simulink model "ExtensionSimulation1var_5"  (R2017b)
settings: Solver=VariableStepAuto  StartTime=0.0  StopTime=60  RelTol=1e-3  EnableMultiTasking=on
values from neighbouring files (symbols this model uses):
  CHNoise = 1e-05    [Extension 1 Variables.mat]    (also in PlotChannelDiscrete.m = 1e-10; PlotChannelsExt.m = 0.0001; SelectivityFunction.m = 0.001)
  nu_gpe = 1    [Extension 1 Variables.mat]
  nu_gpi = 1    [Extension 1 Variables.mat]
  nu_stn = 1    [Extension 1 Variables.mat]
  nu_str = 1    [Extension 1 Variables.mat]
  teta = 0.02    [Extension 1 Variables.mat]
  w_e = 0.9    [Extension 1 Variables.mat]    (also in PlotChannelsExt.m = 1)
  w_g = 1    [Extension 1 Variables.mat]
  w_inh = 0    [Extension 1 Variables.mat]    (also in PlotChannelsExt.m = 0.1)
  w_minus = 1    [Extension 1 Variables.mat]    (also in PlotChannelsExt.m = 1.05)
  w_plus = 0.9    [Extension 1 Variables.mat]    (also in PlotChannelsExt.m = 1)
  w_s = 1    [Extension 1 Variables.mat]    (also in PlotChannelsExt.m)
  w_t = 0.9    [Extension 1 Variables.mat]    (also in PlotChannelsExt.m = 1)
undefined symbols (not defined in the file or in its folder): sigbuilder_block
libraries: fuzblock x25, simulink x8
settings Model: Creator=User  LastModifiedBy=acaso
settings DataIOCC: LimitDataPoints=on
settings OptimizationCC: LifeSpan=inf
settings DebuggingCC: AllowSymbolicDim=off  SFUnexpectedBacktrackingDiag=warning  SFNoUnconditionalDefaultTransitionDiag=warning  SFExecutionAtInitializationDiag=none
settings ModelReferenceCC: PropagateSignalLabelsOutOfModel=off
settings CodeAppCC: StateflowObjectComments=on
settings GRTTargetCC: TargetLangStandard=C89/C90 (ANSI)
settings ConfigComp: CovMetricSettings=dw  CovHtmlReporting=on  CovSaveCumulativeToWorkspaceVar=on  CovSaveSingleToWorkspaceVar=on  CovExternalEMLEnable=off

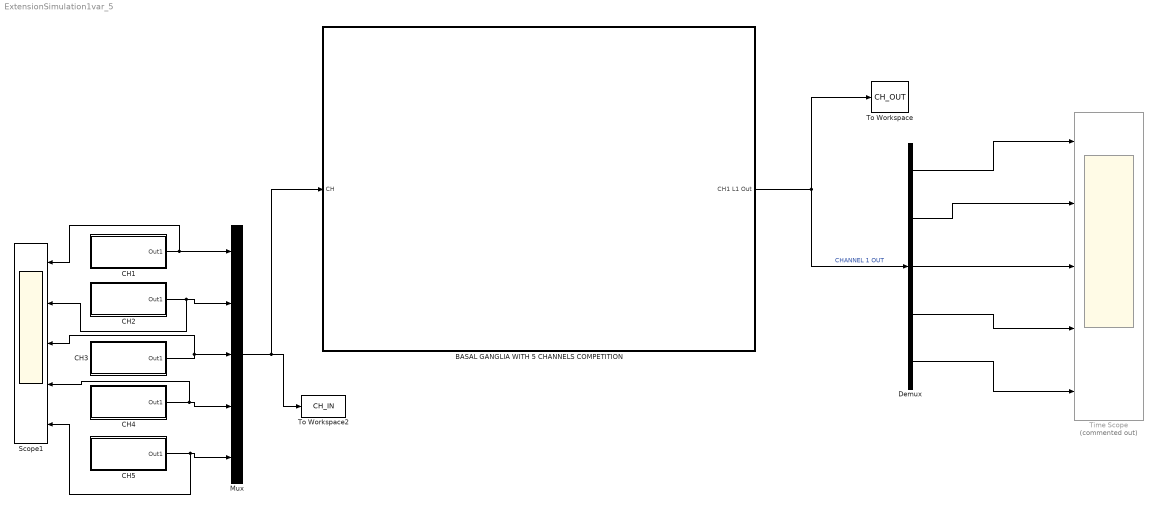
== system ExtensionSimulation1var_5 ==
  BASAL GANGLIA WITH 5 CHANNELS COMPETITION : Subsystem
  "CH1 " : Subsystem
  CH2 : Subsystem
  "CH3 " : Subsystem
  "CH4 " : Subsystem
  "CH5 " : Subsystem
  Demux : Demux  Outputs=5
  Mux : Mux  Inputs=5
  Scope1 : Scope  NumInputPorts=5
  Time Scope : Scope  Commented=on  NumInputPorts=5
  To Workspace : ToWorkspace  VariableName=CH_OUT  SaveFormat=Timeseries  SampleTime=0.1
      settings: Save2DSignal=2-D array (concatenate along first dimension)
  To Workspace2 : ToWorkspace  VariableName=CH_IN  SaveFormat=Timeseries  SampleTime=0.1
  wires:
  BASAL GANGLIA WITH 5 CHANNELS COMPETITION/1(CH1 L1 Out) -> Demux/1, To Workspace/1  "CHANNEL 1 OUT"
  "CH1 "/1(Out1) -> Scope1/1, Mux/1
  "CH3 "/1(Out1) -> Scope1/3, Mux/3
  "CH4 "/1(Out1) -> Scope1/4, Mux/4
  "CH5 "/1(Out1) -> Scope1/5, Mux/5
  Mux/1 -> BASAL GANGLIA WITH 5 CHANNELS COMPETITION/1("CH "), To Workspace2/1
  Demux/1 -> Time Scope/1
  Demux/2 -> Time Scope/2
  Demux/3 -> Time Scope/3
  Demux/4 -> Time Scope/4
  Demux/5 -> Time Scope/5
  CH2/1(Out1) -> Scope1/2, Mux/2

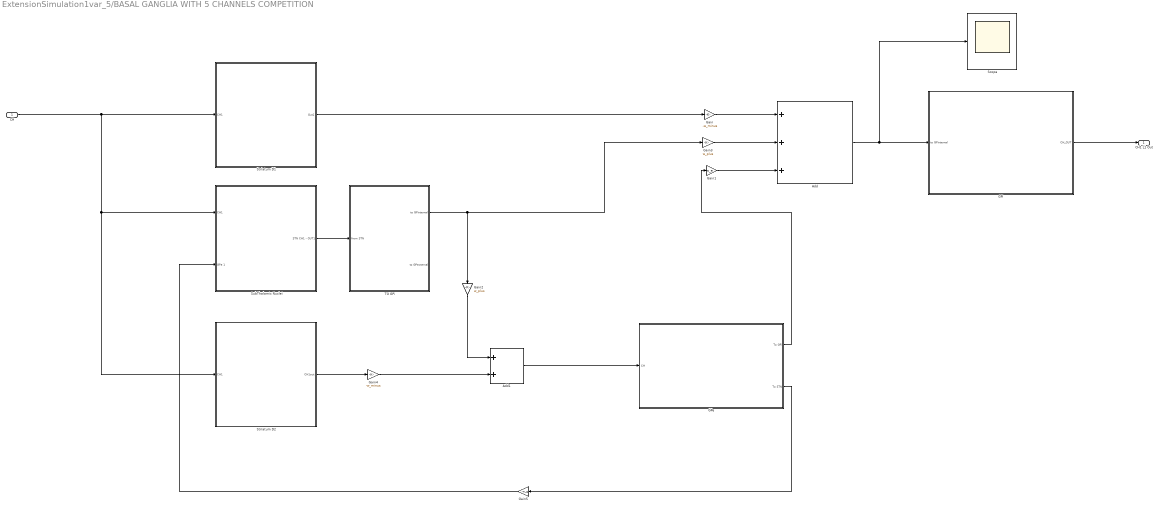
== system ExtensionSimulation1var_5/BASAL GANGLIA WITH 5 CHANNELS COMPETITION ==
  "CH " : Inport
  Add : Sum  Inputs=3
  Add1 : Sum  Inputs=2
  GPe : Subsystem  TreatAsAtomicUnit=on
  GPi : Subsystem
  Gain : Gain  Gain=-w_minus
  Gain1 : Gain  Gain=w_e
  Gain2 : Gain  Gain=w_plus
  Gain3 : Gain  Gain=w_plus
  Gain4 : Gain  Gain=-w_minus
  Gain5 : Gain  Gain=-w_g
  Scope : Scope
  "Striatum D1 " : Subsystem
  Striatum D2 : Subsystem
  SubThalamic Nuclei : Subsystem
  TO GPi : Subsystem
  CH1 L1 Out : Outport
  wires:
  TO GPi/1(to GPinternal) -> Gain2/1, Gain3/1
  GPi/1("CH_OUT ") -> CH1 L1 Out/1
  "CH "/1 -> Striatum D2/1(CH1), SubThalamic Nuclei/1(CH1), "Striatum D1 "/1(CH1)
  "Striatum D1 "/1(Out1) -> Gain/1
  SubThalamic Nuclei/1(STN CH1 - OUT1) -> TO GPi/1("from STN ")
  GPe/1(To GPi) -> Gain1/1
  Gain/1 -> Add/1
  Gain3/1 -> Add/2
  Gain1/1 -> Add/3
  Striatum D2/1(CH1out) -> Gain4/1
  Gain2/1 -> Add1/1
  Gain4/1 -> Add1/2
  Add1/1 -> GPe/1(CH)
  GPe/2(To STN) -> Gain5/1
  Gain5/1 -> SubThalamic Nuclei/2(GPe 1)
  Add/1 -> GPi/1("to GPinternal "), Scope/1

== system ExtensionSimulation1var_5/CH1  ==
  Add : Sum
  Band-Limited White Noise : simulink/Sources/Band-Limited White Noise  Cov=[CHNoise]  Ts=0.1  seed=[23341]
  "CHANNEL1 IN " : Subsystem  Tag=STV Subsys  LoadFcn=sigbuilder_block('load');  StartFcn=sigbuilder_block('start');  StopFcn=sigbuilder_block('stop');  ClipboardFcn=sigbuilder_block('clipboard');  mask(Sigbuilder block){tuvar=[0:10]}
      mask help: Simulink:masks:SigbuilderBlock_MD
      mask init:
      | if ~strcmp(get_param(bdroot(gcbh),'SimulationStatus'),'stopped') tuvar = sigbuilder_block('maskInit'); end
      settings: CopyFcn=sigbuilder_block('copy');  DeleteFcn=sigbuilder_block('delete');  ModelCloseFcn=sigbuilder_block('modelClose');  PreSaveFcn=sigbuilder_block('preSave');  PauseFcn=sigbuilder_block('pause');  ContinueFcn=sigbuilder_block('continue');  NameChangeFcn=sigbuilder_block('namechange');  OpenFcn=sigbuilder_block('open',[5.4 5.4 1141.2 580.8 ]);  CloseFcn=sigbuilder_block('close');
      mask Display: plot(0, 0, 100, 100,[2, 2, 32, 32, 2], [68, 8, 8, 68, 68],[32, 2], [38, 38], [32, 19, 2],[53, 60, 44], [32, 17, 17, 2],[16, 16, 31, 31]);txt = getActiveGroup(gcbh);text(2, 100, txt,'verticalAlignment', 'top');
  Out1 : Outport
  wires:
  Band-Limited White Noise/1 -> Add/2
  Add/1 -> Out1/1
  "CHANNEL1 IN "/1(Signal 1) -> Add/1

== system ExtensionSimulation1var_5/CH2 ==
  Add : Sum
  Band-Limited White Noise : simulink/Sources/Band-Limited White Noise  Cov=[CHNoise]  Ts=0.1  seed=[23341]
  "CHANNEL2 IN " : Subsystem  Tag=STV Subsys  LoadFcn=sigbuilder_block('load');  StartFcn=sigbuilder_block('start');  StopFcn=sigbuilder_block('stop');  ClipboardFcn=sigbuilder_block('clipboard');  mask(Sigbuilder block){tuvar=[0:10]}
      mask help: Simulink:masks:SigbuilderBlock_MD
      mask init:
      | if ~strcmp(get_param(bdroot(gcbh),'SimulationStatus'),'stopped') tuvar = sigbuilder_block('maskInit'); end
      settings: CopyFcn=sigbuilder_block('copy');  DeleteFcn=sigbuilder_block('delete');  ModelCloseFcn=sigbuilder_block('modelClose');  PreSaveFcn=sigbuilder_block('preSave');  PauseFcn=sigbuilder_block('pause');  ContinueFcn=sigbuilder_block('continue');  NameChangeFcn=sigbuilder_block('namechange');  OpenFcn=sigbuilder_block('open',[268.8 5.4 877.8 580.8 ]);  CloseFcn=sigbuilder_block('close');
      mask Display: plot(0, 0, 100, 100,[2, 2, 32, 32, 2], [68, 8, 8, 68, 68],[32, 2], [38, 38], [32, 19, 2],[53, 60, 44], [32, 17, 17, 2],[16, 16, 31, 31]);txt = getActiveGroup(gcbh);text(2, 100, txt,'verticalAlignment', 'top');
  Out1 : Outport
  wires:
  Band-Limited White Noise/1 -> Add/2
  Add/1 -> Out1/1
  "CHANNEL2 IN "/1(Signal 1) -> Add/1

== system ExtensionSimulation1var_5/CH3  ==
  Add : Sum
  Band-Limited White Noise : simulink/Sources/Band-Limited White Noise  Cov=[CHNoise]  Ts=0.1  seed=[23341]
  "CHANNEL2 IN " : Subsystem  Tag=STV Subsys  LoadFcn=sigbuilder_block('load');  StartFcn=sigbuilder_block('start');  StopFcn=sigbuilder_block('stop');  ClipboardFcn=sigbuilder_block('clipboard');  mask(Sigbuilder block){tuvar=[0:10]}
      mask help: Simulink:masks:SigbuilderBlock_MD
      mask init:
      | if ~strcmp(get_param(bdroot(gcbh),'SimulationStatus'),'stopped') tuvar = sigbuilder_block('maskInit'); end
      settings: CopyFcn=sigbuilder_block('copy');  DeleteFcn=sigbuilder_block('delete');  ModelCloseFcn=sigbuilder_block('modelClose');  PreSaveFcn=sigbuilder_block('preSave');  PauseFcn=sigbuilder_block('pause');  ContinueFcn=sigbuilder_block('continue');  NameChangeFcn=sigbuilder_block('namechange');  OpenFcn=sigbuilder_block('open',[5.4 5.4 1141.2 580.8 ]);  CloseFcn=sigbuilder_block('close');
      mask Display: plot(0, 0, 100, 100,[2, 2, 32, 32, 2], [68, 8, 8, 68, 68],[32, 2], [38, 38], [32, 19, 2],[53, 60, 44], [32, 17, 17, 2],[16, 16, 31, 31]);txt = getActiveGroup(gcbh);text(2, 100, txt,'verticalAlignment', 'top');
  Out1 : Outport
  wires:
  Band-Limited White Noise/1 -> Add/2
  Add/1 -> Out1/1
  "CHANNEL2 IN "/3(Signal 2) -> Add/1

== system ExtensionSimulation1var_5/CH4  ==
  Add : Sum
  Band-Limited White Noise : simulink/Sources/Band-Limited White Noise  Cov=[CHNoise]  Ts=0.1  seed=[23341]
  "CHANNEL2 IN " : Subsystem  Tag=STV Subsys  LoadFcn=sigbuilder_block('load');  StartFcn=sigbuilder_block('start');  StopFcn=sigbuilder_block('stop');  ClipboardFcn=sigbuilder_block('clipboard');  mask(Sigbuilder block){tuvar=[0:10]}
      mask help: Simulink:masks:SigbuilderBlock_MD
      mask init:
      | if ~strcmp(get_param(bdroot(gcbh),'SimulationStatus'),'stopped') tuvar = sigbuilder_block('maskInit'); end
      settings: CopyFcn=sigbuilder_block('copy');  DeleteFcn=sigbuilder_block('delete');  ModelCloseFcn=sigbuilder_block('modelClose');  PreSaveFcn=sigbuilder_block('preSave');  PauseFcn=sigbuilder_block('pause');  ContinueFcn=sigbuilder_block('continue');  NameChangeFcn=sigbuilder_block('namechange');  OpenFcn=sigbuilder_block('open',[5.4 5.4 1141.2 580.8 ]);  CloseFcn=sigbuilder_block('close');
      mask Display: plot(0, 0, 100, 100,[2, 2, 32, 32, 2], [68, 8, 8, 68, 68],[32, 2], [38, 38], [32, 19, 2],[53, 60, 44], [32, 17, 17, 2],[16, 16, 31, 31]);txt = getActiveGroup(gcbh);text(2, 100, txt,'verticalAlignment', 'top');
  Out1 : Outport
  wires:
  Band-Limited White Noise/1 -> Add/2
  Add/1 -> Out1/1
  "CHANNEL2 IN "/2(Signal 2) -> Add/1

== system ExtensionSimulation1var_5/CH5  ==
  Add : Sum
  Band-Limited White Noise : simulink/Sources/Band-Limited White Noise  Cov=[CHNoise]  Ts=0.1  seed=[23341]
  "CHANNEL2 IN " : Subsystem  Tag=STV Subsys  LoadFcn=sigbuilder_block('load');  StartFcn=sigbuilder_block('start');  StopFcn=sigbuilder_block('stop');  ClipboardFcn=sigbuilder_block('clipboard');  mask(Sigbuilder block){tuvar=[0:10]}
      mask help: Simulink:masks:SigbuilderBlock_MD
      mask init:
      | if ~strcmp(get_param(bdroot(gcbh),'SimulationStatus'),'stopped') tuvar = sigbuilder_block('maskInit'); end
      settings: CopyFcn=sigbuilder_block('copy');  DeleteFcn=sigbuilder_block('delete');  ModelCloseFcn=sigbuilder_block('modelClose');  PreSaveFcn=sigbuilder_block('preSave');  PauseFcn=sigbuilder_block('pause');  ContinueFcn=sigbuilder_block('continue');  NameChangeFcn=sigbuilder_block('namechange');  OpenFcn=sigbuilder_block('open',[5.4 5.4 1141.2 580.8 ]);  CloseFcn=sigbuilder_block('close');
      mask Display: plot(0, 0, 100, 100,[2, 2, 32, 32, 2], [68, 8, 8, 68, 68],[32, 2], [38, 38], [32, 19, 2],[53, 60, 44], [32, 17, 17, 2],[16, 16, 31, 31]);txt = getActiveGroup(gcbh);text(2, 100, txt,'verticalAlignment', 'top');
  Out1 : Outport
  wires:
  Band-Limited White Noise/1 -> Add/2
  Add/1 -> Out1/1
  "CHANNEL2 IN "/2(Signal 2) -> Add/1

== system ExtensionSimulation1var_5/BASAL GANGLIA WITH 5 CHANNELS COMPETITION/GPe ==
  CH : Inport
  GPe CH1 : Subsystem
  To GPi : Outport
  To STN : Outport  Port=2
  wires:
  CH/1 -> GPe CH1/1(In)
  GPe CH1/1(To GPi) -> To GPi/1
  GPe CH1/2(To STN) -> To STN/1

== system ExtensionSimulation1var_5/BASAL GANGLIA WITH 5 CHANNELS COMPETITION/GPi ==
  "to GPinternal " : Inport
  GPinternal : Subsystem
  "CH_OUT " : Outport
  wires:
  "to GPinternal "/1 -> GPinternal/1("to GPinternal ")
  GPinternal/1(To Thal) -> "CH_OUT "/1

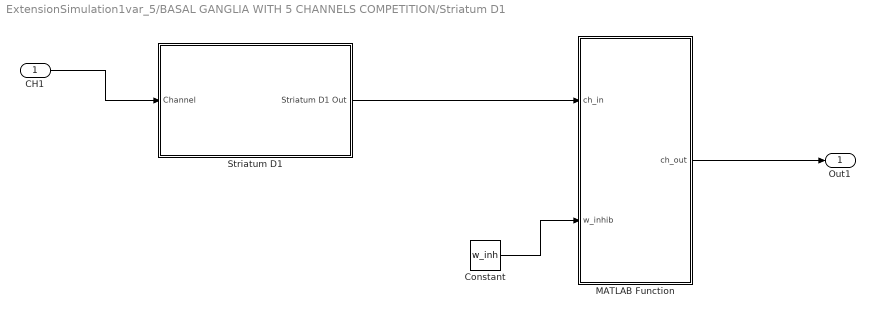
== system ExtensionSimulation1var_5/BASAL GANGLIA WITH 5 CHANNELS COMPETITION/Striatum D1  ==
  CH1 : Inport
  Constant : Constant  Value=w_inh
  MATLAB Function : MATLAB Function  TreatAsAtomicUnit=on
  "Striatum D1 " : Subsystem
  Out1 : Outport
  wires:
  CH1/1 -> "Striatum D1 "/1(Channel)
  "Striatum D1 "/1(Striatum D1 Out) -> MATLAB Function/1(ch_in)
  Constant/1 -> MATLAB Function/2(w_inhib)
  MATLAB Function/1(ch_out) -> Out1/1

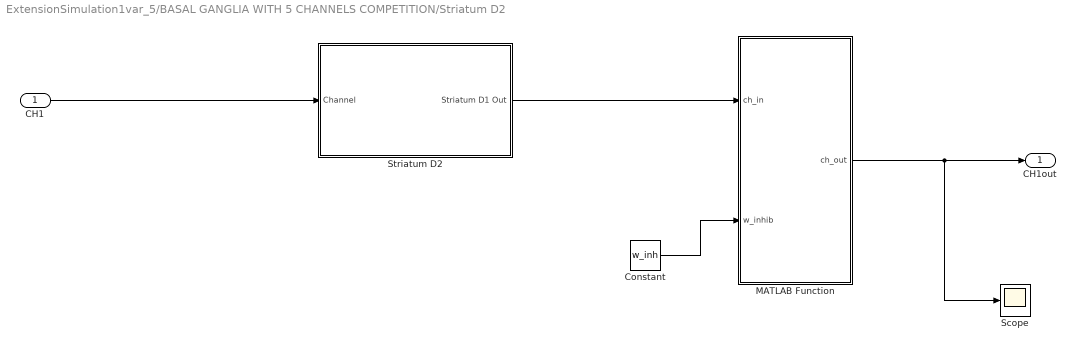
== system ExtensionSimulation1var_5/BASAL GANGLIA WITH 5 CHANNELS COMPETITION/Striatum D2 ==
  CH1 : Inport
  Constant : Constant  Value=w_inh
  MATLAB Function : MATLAB Function  TreatAsAtomicUnit=on
  Scope : Scope
  "Striatum D2 " : Subsystem
  CH1out : Outport
  wires:
  MATLAB Function/1(ch_out) -> Scope/1, CH1out/1
  CH1/1 -> "Striatum D2 "/1(Channel)
  "Striatum D2 "/1(Striatum D1 Out) -> MATLAB Function/1(ch_in)
  Constant/1 -> MATLAB Function/2(w_inhib)

== system ExtensionSimulation1var_5/BASAL GANGLIA WITH 5 CHANNELS COMPETITION/SubThalamic Nuclei ==
  CH1 : Inport
  GPe 1 : Inport  Port=2
  "SubThalamic Nucleus (STN) " : Subsystem
  STN CH1 - OUT1 : Outport
  wires:
  CH1/1 -> "SubThalamic Nucleus (STN) "/1(Channel)
  GPe 1/1 -> "SubThalamic Nucleus (STN) "/2(GPe Inp)
  "SubThalamic Nucleus (STN) "/1(STN Out1) -> STN CH1 - OUT1/1

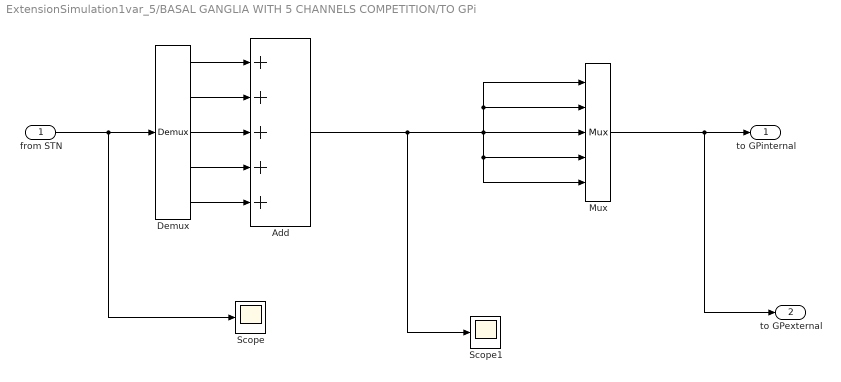
== system ExtensionSimulation1var_5/BASAL GANGLIA WITH 5 CHANNELS COMPETITION/TO GPi ==
  "from STN " : Inport
  Add : Sum  Inputs=5
  Demux : Demux  Outputs=5
  Mux : Mux  Inputs=5
  Scope : Scope
  Scope1 : Scope
  to GPinternal : Outport
  to GPexternal : Outport  Port=2
  wires:
  "from STN "/1 -> Scope/1, Demux/1
  Demux/1 -> Add/1
  Demux/2 -> Add/2
  Demux/3 -> Add/3
  Demux/4 -> Add/4
  Demux/5 -> Add/5
  Add/1 -> Scope1/1, Mux/1, Mux/2, Mux/3, Mux/4, Mux/5
  Mux/1 -> to GPexternal/1, to GPinternal/1

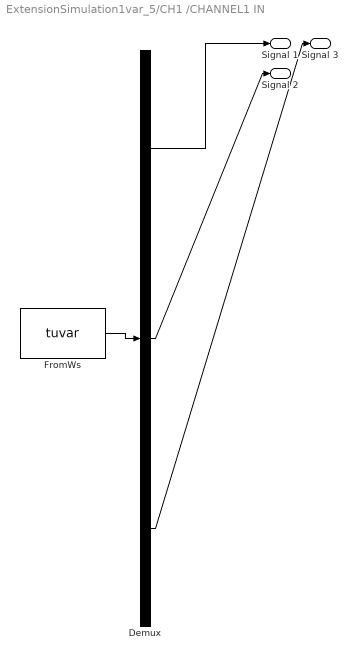
== system ExtensionSimulation1var_5/CH1 /CHANNEL1 IN  ==
  Demux : Demux  Tag=STV Demux  Outputs=3
  FromWs : FromWorkspace  Tag=STV FromWs  VariableName=tuvar  SampleTime=0
      SigBuilderData=|
      | common.afterFinalStr = 'Extrapolate'
      | common.sampleTime = 0
      | dataSet.timeRange = [0 35]
      | dataSet.name = 'Group 1'
      | sbobj.Groups.Name = 'Group 1'
      | sbobj.Groups.Signals(1).Name = 'Signal 1'
      | sbobj.Groups.Signals(1).XData = [0 5 5 10 10 15 15 20 20 25 25 35]
      | sbobj.Groups.Signals(1).YData = [-0.002 -0.002 0.4 0.402 0.598 0.598 0.898 0.898 0.4 0.4 -0.002 -0.002]
      | sbobj.Groups.Signals(2).Name = 'Signal 2'
      | sbobj.Groups.Signals(2).XData = [0 10 10 19.95 19.95 35]
      | sbobj.Groups.Signals(2).YData = [0 0 1 1 0 0]
      | sbobj.Groups.Signals(3).Name = 'Signal 3'
      | sbobj.Groups.Signals(3).XData = [0 0.124999063463 0.124999063463 0.554655534638 0.554655534638 1.75407532206 1.75407532206 2.41531933083 2.41531933083 3.35183646647 3.35183646647 3.98652733627 3.98652733627 4.3969208728 4.3969208728 4.71706282774 4.71706282774 5.10813469216 5.10813469216 5.17468809149 5.17468809149 5.50352781473 5.50352781473 5.53254229218 5.53254229218 5.75747882155 5.75747882155 5.7790923367 5.7790923367 6.49117968939 6.49117968939 6.6868703376 6.6868703376 7.30742292982 7.30742292982 7.50631415349 7.50631415349 7.6881348016 7.6881348016 9.03231176435 9.03231176435 9.7159692583 9.7159692583 10.4639345253 10.4639345253 10.6657932981 10.6657932981 10.750362424 10.750362424 11.2832475767 11.2832475767 11.4071452565 11.4071452565 11.6034206364 11.6034206364 14.1051029573 14.1051029573 14.3587102932 14.3587102932 14.8336712879 14.8336712879 14.8775455245 14.8775455245 18.2610827825 18.2610827825 18.6466921096 18.6466921096 19.0752915872 19.0752915872 19.4625609227 19.4625609227 19.5931395957 19.5931395957 20.1590093787 20.1590093787 20.2802112412 20.2802112412 20.6562808333 20.6562808333 22.3217052823 22.3217052823 23.1906978252 23.1906978252 23.3537304902 23.3537304902 23.7275469646 23.7275469646 24.6671175842 24.6671175842 25.2048713101 25.2048713101 25.4541640524 25.4541640524 26.2799578436 26.2799578436 26.4315744674 26.4315744674 27.1392309495 27.1392309495 27.1823235313 27.1823235313 27.8387310207 27.8387310207 27.9723440417 27.9723440417 28.8062432156 28.8062432156 29.4295126023 29.4295126023 30.62733745 30.62733745 30.9029795381 30.9029795381 31.093343901 31.093343901 31.3953692022 31.3953692022 31.8223455306 31.8223455306 32.0420301508 32.0420301508 32.2592575676 32.2592575676 32.4528123061 32.4528123061 32.6792583725 32.6792583725 32.7074514334 32.7074514334 33.4903176591 33.4903176591 33.6620689128 33.6620689128 35]
      | sbobj.Groups.Signals(3).YData = [0 0 1 1 0 0 1 1 0 0 1 1 0 0 1 1 0 0 1 1 0 0 1 1 0 0 1 1 0 0 1 1 0 0 1 1 0 0 1 1 0 0 1 1 0 0 1 1 0 0 1 1 0 0 1 1 0 0 1 1 0 0 1 1 0 0 1 1 0 0 1 1 0 0 1 1 0 0 1 1 0 0 1 1 0 0 1 1 0 0 1 1 0 0 1 1 0 0 1 1 0 0 1 1 0 0 1 1 0 0 1 1 0 0 1 1 0 0 1 1 0 0 1 1 0 0 1 1 0 0 1 1 0 0]
      | sbobj.Groups.TimeRange = [0 35]
  Signal 1 : Outport  Tag=STV Outport
  Signal 2 : Outport  Tag=STV Outport  Port=2
  Signal 3 : Outport  Tag=STV Outport  Port=3
  wires:
  Demux/1 -> Signal 1/1
  FromWs/1 -> Demux/1
  Demux/2 -> Signal 2/1
  Demux/3 -> Signal 3/1

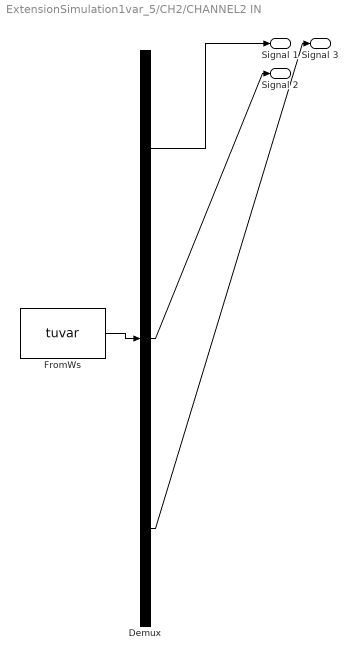
== system ExtensionSimulation1var_5/CH2/CHANNEL2 IN  ==
  Demux : Demux  Tag=STV Demux  Outputs=3
  FromWs : FromWorkspace  Tag=STV FromWs  VariableName=tuvar  SampleTime=0
      SigBuilderData=|
      | common.afterFinalStr = 'Extrapolate'
      | common.sampleTime = 0
      | dataSet.timeRange = [0 35]
      | dataSet.name = 'Group 1'
      | sbobj.Groups.Name = 'Group 1'
      | sbobj.Groups.Signals(1).Name = 'Signal 1'
      | sbobj.Groups.Signals(1).XData = [0 10 10 15.05 15.05 20 20 24.95 24.95 30 30 35]
      | sbobj.Groups.Signals(1).YData = [-0.002 -0.002 0.40108 0.402 0.598 0.598 0.898 0.898 0.405 0.405 -0.002 -0.002]
      | sbobj.Groups.Signals(2).Name = 'Signal 2'
      | sbobj.Groups.Signals(2).XData = [0 15 15 25.05 25.05 35]
      | sbobj.Groups.Signals(2).YData = [0 0 1 1 0 0]
      | sbobj.Groups.Signals(3).Name = 'Signal 3'
      | sbobj.Groups.Signals(3).XData = [0 0.572735490782 0.572735490782 1.63615076232 1.63615076232 1.66717917967 1.66717917967 1.88600403363 1.88600403363 2.25354807472 2.25354807472 2.47722553518 ... (160 elements, 1x160)]
      | sbobj.Groups.Signals(3).YData = [0 0 1 1 0 0 1 1 0 0 1 1 0 0 1 1 0 0 1 1 0 0 1 1 0 0 1 1 0 0 1 1 0 0 1 1 0 0 1 1 0 0 1 1 0 0 1 1 0 0 1 1 0 0 1 1 0 0 1 1 0 0 1 1 0 0 1 1 0 0 1 1 0 0 1 1 0 0 1 1 0 0 1 1 0 0 1 1 0 0 1 1 0 0 1 1 0 0 1 1 0 0 1 1 0 0 1 1 0 0 1 1 0 0 1 1 0 0 1 1 0 0 1 1 0 0 1 1 0 0 1 1 0 0 1 1 0 0 1 1 0 0 1 1 0 0 1 1 0 0 1 1 0 0 1 1 0 0 1 1]
      | sbobj.Groups.TimeRange = [0 35]
  Signal 1 : Outport  Tag=STV Outport
  Signal 2 : Outport  Tag=STV Outport  Port=2
  Signal 3 : Outport  Tag=STV Outport  Port=3
  wires:
  Demux/1 -> Signal 1/1
  FromWs/1 -> Demux/1
  Demux/2 -> Signal 2/1
  Demux/3 -> Signal 3/1

== system ExtensionSimulation1var_5/CH3 /CHANNEL2 IN  ==
  Demux : Demux  Tag=STV Demux  Outputs=3
  FromWs : FromWorkspace  Tag=STV FromWs  VariableName=tuvar  SampleTime=0
      SigBuilderData=|
      | common.afterFinalStr = 'Extrapolate'
      | common.sampleTime = 0
      | dataSet.timeRange = [0 35]
      | dataSet.name = 'Group 1'
      | sbobj.Groups.Name = 'Group 1'
      | sbobj.Groups.Signals(1).Name = 'Signal 3'
      | sbobj.Groups.Signals(1).XData = [0 35]
      | sbobj.Groups.Signals(1).YData = [0.195 0.195]
      | sbobj.Groups.Signals(2).Name = 'Signal 1'
      | sbobj.Groups.Signals(2).XData = [0 16.35 16.35 32.85 32.85 35]
      | sbobj.Groups.Signals(2).YData = [0 0 1 1 0 0]
      | sbobj.Groups.Signals(3).Name = 'Signal 2'
      | sbobj.Groups.Signals(3).XData = [0 5 5 10 10 15 15 20 20 25 25 30 30 35]
      | sbobj.Groups.Signals(3).YData = [1 1 0.72 0.72 0.24 0.24 -0.02 -0.02 0.36 0.36 0.86 0.86 1.12 1.12]
      | sbobj.Groups.TimeRange = [0 35]
  Signal 3 : Outport  Tag=STV Outport
  Signal 1 : Outport  Tag=STV Outport  Port=2
  Signal 2 : Outport  Tag=STV Outport  Port=3
  wires:
  FromWs/1 -> Demux/1
  Demux/1 -> Signal 3/1
  Demux/2 -> Signal 1/1
  Demux/3 -> Signal 2/1

== system ExtensionSimulation1var_5/CH4 /CHANNEL2 IN  ==
  Demux : Demux  Tag=STV Demux  Outputs=2
  FromWs : FromWorkspace  Tag=STV FromWs  VariableName=tuvar  SampleTime=0
      SigBuilderData=|
      | common.afterFinalStr = 'Extrapolate'
      | common.sampleTime = 0
      | dataSet.timeRange = [0 35]
      | dataSet.name = 'Group 1'
      | sbobj.Groups.Name = 'Group 1'
      | sbobj.Groups.Signals(1).Name = 'Signal 1'
      | sbobj.Groups.Signals(1).XData = [0 28.15 28.15 31.75 31.75 35]
      | sbobj.Groups.Signals(1).YData = [0 0 1 1 0 0]
      | sbobj.Groups.Signals(2).Name = 'Signal 2'
      | sbobj.Groups.Signals(2).XData = [0 5 5 10 10 15 15 20 20 25 25 30 30 35]
      | sbobj.Groups.Signals(2).YData = [0 0.9 0.02 1 0.48 0.26 0.62 1 0.74 0.54 0.28 0.14 0.8 1]
      | sbobj.Groups.TimeRange = [0 35]
  Signal 1 : Outport  Tag=STV Outport
  Signal 2 : Outport  Tag=STV Outport  Port=2
  wires:
  FromWs/1 -> Demux/1
  Demux/1 -> Signal 1/1
  Demux/2 -> Signal 2/1

== system ExtensionSimulation1var_5/CH5 /CHANNEL2 IN  ==
  Demux : Demux  Tag=STV Demux  Outputs=2
  FromWs : FromWorkspace  Tag=STV FromWs  VariableName=tuvar  SampleTime=0
      SigBuilderData=|
      | common.afterFinalStr = 'Extrapolate'
      | common.sampleTime = 0
      | dataSet.timeRange = [0 35]
      | dataSet.name = 'Group 1'
      | sbobj.Groups.Name = 'Group 1'
      | sbobj.Groups.Signals(1).Name = 'Signal 1'
      | sbobj.Groups.Signals(1).XData = [0 29.7 29.7 33.95 33.95 35]
      | sbobj.Groups.Signals(1).YData = [0.051 0.051 0.78 0.78 0.049 0.049]
      | sbobj.Groups.Signals(2).Name = 'Signal 2'
      | sbobj.Groups.Signals(2).XData = [0 4 8 12 16 20 24 29.25 29.25 35]
      | sbobj.Groups.Signals(2).YData = [0.737667139546 0.375 0.625 0.1 0.518765239859 0.3 0.345 0.245 0.635 0.25]
      | sbobj.Groups.TimeRange = [0 35]
  Signal 1 : Outport  Tag=STV Outport
  Signal 2 : Outport  Tag=STV Outport  Port=2
  wires:
  FromWs/1 -> Demux/1
  Demux/1 -> Signal 1/1
  Demux/2 -> Signal 2/1

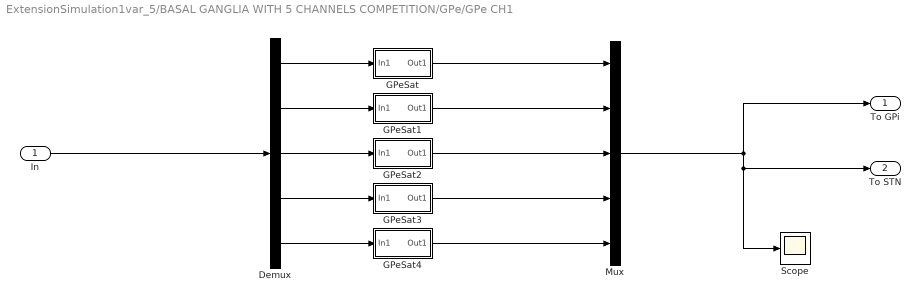
== system ExtensionSimulation1var_5/BASAL GANGLIA WITH 5 CHANNELS COMPETITION/GPe/GPe CH1 ==
  In : Inport
  Demux : Demux  Outputs=5
  GPeSat : Subsystem
  GPeSat1 : Subsystem
  GPeSat2 : Subsystem
  GPeSat3 : Subsystem
  GPeSat4 : Subsystem
  Mux : Mux  Inputs=5
  Scope : Scope
  To GPi : Outport
  To STN : Outport  Port=2
  wires:
  Mux/1 -> To STN/1, Scope/1, To GPi/1
  Demux/1 -> GPeSat/1(In1)
  GPeSat/1(Out1) -> Mux/1
  Demux/2 -> GPeSat1/1(In1)
  GPeSat1/1(Out1) -> Mux/2
  Demux/3 -> GPeSat2/1(In1)
  GPeSat2/1(Out1) -> Mux/3
  Demux/4 -> GPeSat3/1(In1)
  GPeSat3/1(Out1) -> Mux/4
  Demux/5 -> GPeSat4/1(In1)
  GPeSat4/1(Out1) -> Mux/5
  In/1 -> Demux/1

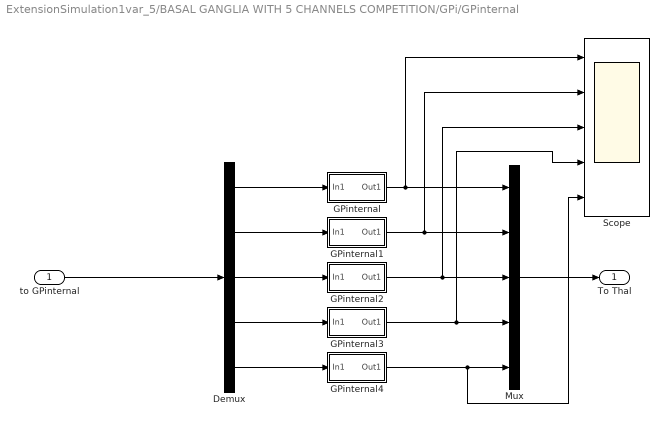
== system ExtensionSimulation1var_5/BASAL GANGLIA WITH 5 CHANNELS COMPETITION/GPi/GPinternal ==
  "to GPinternal " : Inport
  Demux : Demux  Outputs=5
  GPinternal : Subsystem
  GPinternal1 : Subsystem
  GPinternal2 : Subsystem
  GPinternal3 : Subsystem
  GPinternal4 : Subsystem
  Mux : Mux  Inputs=5
  Scope : Scope  NumInputPorts=5
  To Thal : Outport
  wires:
  Demux/1 -> GPinternal/1(In1)
  GPinternal/1(Out1) -> Mux/1, Scope/1
  Demux/2 -> GPinternal1/1(In1)
  Demux/3 -> GPinternal2/1(In1)
  GPinternal2/1(Out1) -> Scope/3, Mux/3
  Demux/4 -> GPinternal3/1(In1)
  GPinternal3/1(Out1) -> Scope/4, Mux/4
  Demux/5 -> GPinternal4/1(In1)
  GPinternal4/1(Out1) -> Scope/5, Mux/5
  "to GPinternal "/1 -> Demux/1
  Mux/1 -> To Thal/1
  GPinternal1/1(Out1) -> Scope/2, Mux/2

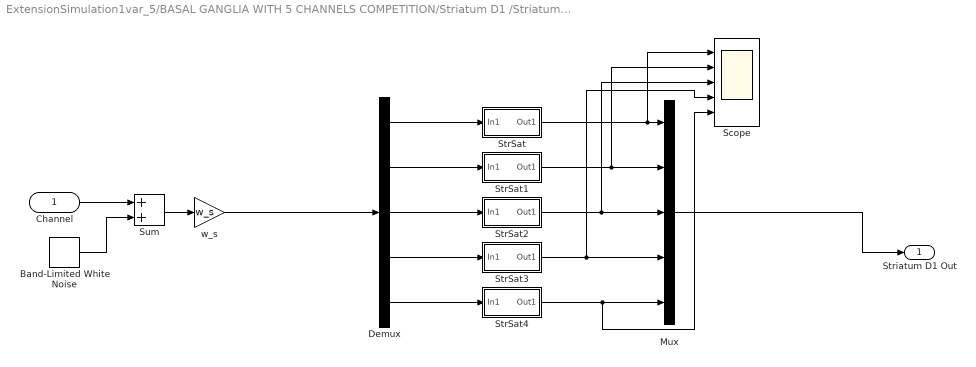
== system ExtensionSimulation1var_5/BASAL GANGLIA WITH 5 CHANNELS COMPETITION/Striatum D1 /Striatum D1  ==
  Channel : Inport
  Band-Limited White Noise : simulink/Sources/Band-Limited White Noise  Cov=[0]  Ts=0.1  seed=[23341]
  Demux : Demux  Outputs=5
  Mux : Mux  Inputs=5
  Scope : Scope  NumInputPorts=5
  StrSat : Subsystem
  StrSat1 : Subsystem
  StrSat2 : Subsystem
  StrSat3 : Subsystem
  StrSat4 : Subsystem
  Sum : Sum
  w_s : Gain  Gain=w_s
  Striatum D1 Out : Outport
  wires:
  Channel/1 -> Sum/1
  Sum/1 -> w_s/1
  Mux/1 -> Striatum D1 Out/1
  Band-Limited White Noise/1 -> Sum/2
  Demux/1 -> StrSat/1(In1)
  StrSat/1(Out1) -> Scope/1, Mux/1
  Demux/2 -> StrSat1/1(In1)
  StrSat1/1(Out1) -> Scope/2, Mux/2
  Demux/3 -> StrSat2/1(In1)
  StrSat2/1(Out1) -> Scope/3, Mux/3
  Demux/4 -> StrSat3/1(In1)
  StrSat3/1(Out1) -> Scope/4, Mux/4
  Demux/5 -> StrSat4/1(In1)
  w_s/1 -> Demux/1
  StrSat4/1(Out1) -> Scope/5, Mux/5

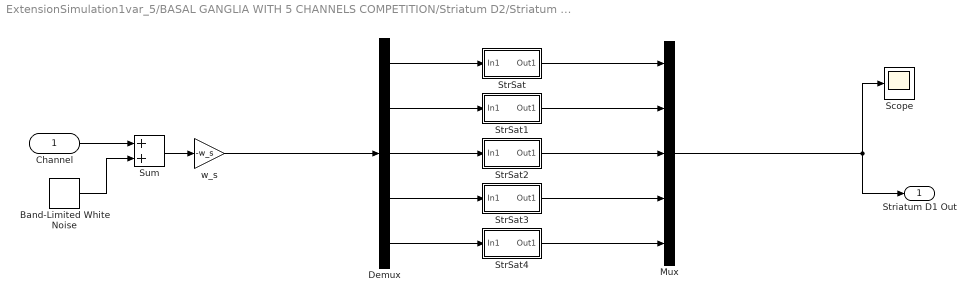
== system ExtensionSimulation1var_5/BASAL GANGLIA WITH 5 CHANNELS COMPETITION/Striatum D2/Striatum D2  ==
  Channel : Inport
  Band-Limited White Noise : simulink/Sources/Band-Limited White Noise  Cov=[0]  Ts=0.1  seed=[23341]
  Demux : Demux  Outputs=5
  Mux : Mux  Inputs=5
  Scope : Scope
  StrSat : Subsystem
  StrSat1 : Subsystem
  StrSat2 : Subsystem
  StrSat3 : Subsystem
  StrSat4 : Subsystem
  Sum : Sum
  w_s : Gain  Gain=-w_s
  Striatum D1 Out : Outport
  wires:
  Channel/1 -> Sum/1
  Sum/1 -> w_s/1
  Mux/1 -> Striatum D1 Out/1, Scope/1
  Band-Limited White Noise/1 -> Sum/2
  Demux/1 -> StrSat/1(In1)
  StrSat/1(Out1) -> Mux/1
  Demux/2 -> StrSat1/1(In1)
  StrSat1/1(Out1) -> Mux/2
  Demux/3 -> StrSat2/1(In1)
  StrSat2/1(Out1) -> Mux/3
  Demux/4 -> StrSat3/1(In1)
  StrSat3/1(Out1) -> Mux/4
  Demux/5 -> StrSat4/1(In1)
  StrSat4/1(Out1) -> Mux/5
  w_s/1 -> Demux/1

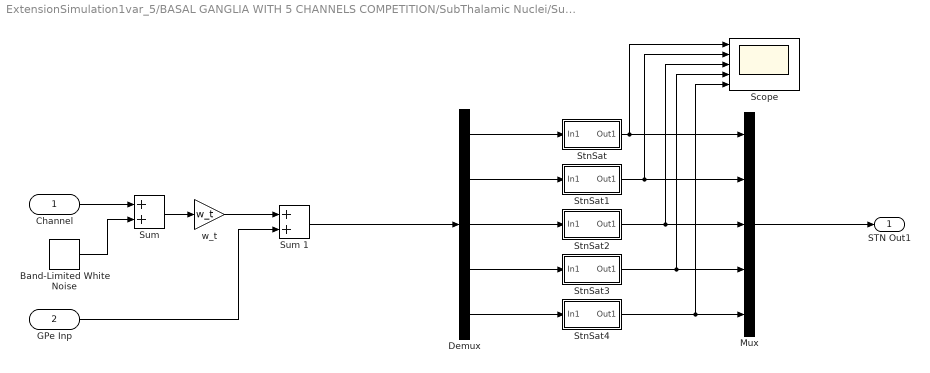
== system ExtensionSimulation1var_5/BASAL GANGLIA WITH 5 CHANNELS COMPETITION/SubThalamic Nuclei/SubThalamic Nucleus (STN)  ==
  Channel : Inport
  GPe Inp : Inport  Port=2
  Band-Limited White Noise : simulink/Sources/Band-Limited White Noise  Cov=[0]  Ts=0.1  seed=[23341]
  Demux : Demux  Outputs=5
  Mux : Mux  Inputs=5
  Scope : Scope  NumInputPorts=5
  StnSat : Subsystem
  StnSat1 : Subsystem
  StnSat2 : Subsystem
  StnSat3 : Subsystem
  StnSat4 : Subsystem
  "Sum " : Sum
  Sum 1 : Sum
  w_t : Gain  Gain=w_t
  STN Out1 : Outport
  wires:
  w_t/1 -> Sum 1/1
  Channel/1 -> "Sum "/1
  Band-Limited White Noise/1 -> "Sum "/2
  "Sum "/1 -> w_t/1
  GPe Inp/1 -> Sum 1/2
  Mux/1 -> STN Out1/1
  Demux/1 -> StnSat/1(In1)
  Demux/2 -> StnSat1/1(In1)
  StnSat1/1(Out1) -> Scope/2, Mux/2
  Demux/3 -> StnSat2/1(In1)
  StnSat2/1(Out1) -> Scope/3, Mux/3
  Demux/4 -> StnSat3/1(In1)
  StnSat3/1(Out1) -> Scope/4, Mux/4
  Demux/5 -> StnSat4/1(In1)
  StnSat4/1(Out1) -> Scope/5, Mux/5
  Sum 1/1 -> Demux/1
  StnSat/1(Out1) -> Scope/1, Mux/1

== system ExtensionSimulation1var_5/BASAL GANGLIA WITH 5 CHANNELS COMPETITION/GPe/GPe CH1/GPeSat ==
  In1 : Inport
  Fcn : Fcn  Expr=u^(1/nu_gpe)
  "Leaky-Integrator Striatum D1 " : ZeroPole  Zeros=[]  Poles=[-1/teta]  Gain=[1.5/teta]
  Sigmoidal MF : fuzblock/Membership  Functions/Sigmoidal MF  a=alpha_gpe  c=beta_gpe
      settings: SourceProductName=Fuzzy Logic Toolbox  SourceProductBaseCode=FL
  Out1 : Outport
  wires:
  Fcn/1 -> Out1/1
  Sigmoidal MF/1 -> Fcn/1
  "Leaky-Integrator Striatum D1 "/1 -> Sigmoidal MF/1
  In1/1 -> "Leaky-Integrator Striatum D1 "/1

== system ExtensionSimulation1var_5/BASAL GANGLIA WITH 5 CHANNELS COMPETITION/GPe/GPe CH1/GPeSat1 ==
  In1 : Inport
  Fcn : Fcn  Expr=u^(1/nu_gpe)
  "Leaky-Integrator Striatum D1 " : ZeroPole  Zeros=[]  Poles=[-1/teta]  Gain=[1.5/teta]
  Sigmoidal MF : fuzblock/Membership  Functions/Sigmoidal MF  a=alpha_gpe  c=beta_gpe
      settings: SourceProductName=Fuzzy Logic Toolbox  SourceProductBaseCode=FL
  Out1 : Outport
  wires:
  Fcn/1 -> Out1/1
  Sigmoidal MF/1 -> Fcn/1
  "Leaky-Integrator Striatum D1 "/1 -> Sigmoidal MF/1
  In1/1 -> "Leaky-Integrator Striatum D1 "/1

== system ExtensionSimulation1var_5/BASAL GANGLIA WITH 5 CHANNELS COMPETITION/GPe/GPe CH1/GPeSat2 ==
  In1 : Inport
  Fcn : Fcn  Expr=u^(1/nu_gpe)
  "Leaky-Integrator Striatum D1 " : ZeroPole  Zeros=[]  Poles=[-1/teta]  Gain=[1.5/teta]
  Sigmoidal MF : fuzblock/Membership  Functions/Sigmoidal MF  a=alpha_gpe  c=beta_gpe
      settings: SourceProductName=Fuzzy Logic Toolbox  SourceProductBaseCode=FL
  Out1 : Outport
  wires:
  Fcn/1 -> Out1/1
  Sigmoidal MF/1 -> Fcn/1
  "Leaky-Integrator Striatum D1 "/1 -> Sigmoidal MF/1
  In1/1 -> "Leaky-Integrator Striatum D1 "/1

== system ExtensionSimulation1var_5/BASAL GANGLIA WITH 5 CHANNELS COMPETITION/GPe/GPe CH1/GPeSat3 ==
  In1 : Inport
  Fcn : Fcn  Expr=u^(1/nu_gpe)
  "Leaky-Integrator Striatum D1 " : ZeroPole  Zeros=[]  Poles=[-1/teta]  Gain=[1.5/teta]
  Sigmoidal MF : fuzblock/Membership  Functions/Sigmoidal MF  a=alpha_gpe  c=beta_gpe
      settings: SourceProductName=Fuzzy Logic Toolbox  SourceProductBaseCode=FL
  Out1 : Outport
  wires:
  Fcn/1 -> Out1/1
  Sigmoidal MF/1 -> Fcn/1
  "Leaky-Integrator Striatum D1 "/1 -> Sigmoidal MF/1
  In1/1 -> "Leaky-Integrator Striatum D1 "/1

== system ExtensionSimulation1var_5/BASAL GANGLIA WITH 5 CHANNELS COMPETITION/GPe/GPe CH1/GPeSat4 ==
  In1 : Inport
  Fcn : Fcn  Expr=u^(1/nu_gpe)
  "Leaky-Integrator Striatum D1 " : ZeroPole  Zeros=[]  Poles=[-1/teta]  Gain=[1.5/teta]
  Sigmoidal MF : fuzblock/Membership  Functions/Sigmoidal MF  a=alpha_gpe  c=beta_gpe
      settings: SourceProductName=Fuzzy Logic Toolbox  SourceProductBaseCode=FL
  Out1 : Outport
  wires:
  Fcn/1 -> Out1/1
  Sigmoidal MF/1 -> Fcn/1
  "Leaky-Integrator Striatum D1 "/1 -> Sigmoidal MF/1
  In1/1 -> "Leaky-Integrator Striatum D1 "/1

== system ExtensionSimulation1var_5/BASAL GANGLIA WITH 5 CHANNELS COMPETITION/GPi/GPinternal/GPinternal ==
  In1 : Inport
  Fcn : Fcn  Expr=u^(1/nu_gpi)
  "Leaky-Integrator Striatum D1 " : ZeroPole  Zeros=[]  Poles=[-1/teta]  Gain=[1.5/teta]
  Sigmoidal MF : fuzblock/Membership  Functions/Sigmoidal MF  a=alpha_gpi  c=beta_gpi
      settings: SourceProductName=Fuzzy Logic Toolbox  SourceProductBaseCode=FL
  Out1 : Outport
  wires:
  Fcn/1 -> Out1/1
  Sigmoidal MF/1 -> Fcn/1
  "Leaky-Integrator Striatum D1 "/1 -> Sigmoidal MF/1
  In1/1 -> "Leaky-Integrator Striatum D1 "/1

== system ExtensionSimulation1var_5/BASAL GANGLIA WITH 5 CHANNELS COMPETITION/GPi/GPinternal/GPinternal1 ==
  In1 : Inport
  Fcn : Fcn  Expr=u^(1/nu_gpi)
  "Leaky-Integrator Striatum D1 " : ZeroPole  Zeros=[]  Poles=[-1/teta]  Gain=[1.5/teta]
  Sigmoidal MF : fuzblock/Membership  Functions/Sigmoidal MF  a=alpha_gpi  c=beta_gpi
      settings: SourceProductName=Fuzzy Logic Toolbox  SourceProductBaseCode=FL
  Out1 : Outport
  wires:
  Fcn/1 -> Out1/1
  Sigmoidal MF/1 -> Fcn/1
  "Leaky-Integrator Striatum D1 "/1 -> Sigmoidal MF/1
  In1/1 -> "Leaky-Integrator Striatum D1 "/1

== system ExtensionSimulation1var_5/BASAL GANGLIA WITH 5 CHANNELS COMPETITION/GPi/GPinternal/GPinternal2 ==
  In1 : Inport
  Fcn : Fcn  Expr=u^(1/nu_gpi)
  "Leaky-Integrator Striatum D1 " : ZeroPole  Zeros=[]  Poles=[-1/teta]  Gain=[1.5/teta]
  Sigmoidal MF : fuzblock/Membership  Functions/Sigmoidal MF  a=alpha_gpi  c=beta_gpi
      settings: SourceProductName=Fuzzy Logic Toolbox  SourceProductBaseCode=FL
  Out1 : Outport
  wires:
  Fcn/1 -> Out1/1
  Sigmoidal MF/1 -> Fcn/1
  "Leaky-Integrator Striatum D1 "/1 -> Sigmoidal MF/1
  In1/1 -> "Leaky-Integrator Striatum D1 "/1

== system ExtensionSimulation1var_5/BASAL GANGLIA WITH 5 CHANNELS COMPETITION/GPi/GPinternal/GPinternal3 ==
  In1 : Inport
  Fcn : Fcn  Expr=u^(1/nu_gpi)
  "Leaky-Integrator Striatum D1 " : ZeroPole  Zeros=[]  Poles=[-1/teta]  Gain=[1.5/teta]
  Sigmoidal MF : fuzblock/Membership  Functions/Sigmoidal MF  a=alpha_gpi  c=beta_gpi
      settings: SourceProductName=Fuzzy Logic Toolbox  SourceProductBaseCode=FL
  Out1 : Outport
  wires:
  Fcn/1 -> Out1/1
  Sigmoidal MF/1 -> Fcn/1
  "Leaky-Integrator Striatum D1 "/1 -> Sigmoidal MF/1
  In1/1 -> "Leaky-Integrator Striatum D1 "/1

== system ExtensionSimulation1var_5/BASAL GANGLIA WITH 5 CHANNELS COMPETITION/GPi/GPinternal/GPinternal4 ==
  In1 : Inport
  Fcn : Fcn  Expr=u^(1/nu_gpi)
  "Leaky-Integrator Striatum D1 " : ZeroPole  Zeros=[]  Poles=[-1/teta]  Gain=[1.5/teta]
  Sigmoidal MF : fuzblock/Membership  Functions/Sigmoidal MF  a=alpha_gpi  c=beta_gpi
      settings: SourceProductName=Fuzzy Logic Toolbox  SourceProductBaseCode=FL
  Out1 : Outport
  wires:
  Fcn/1 -> Out1/1
  Sigmoidal MF/1 -> Fcn/1
  "Leaky-Integrator Striatum D1 "/1 -> Sigmoidal MF/1
  In1/1 -> "Leaky-Integrator Striatum D1 "/1

== system ExtensionSimulation1var_5/BASAL GANGLIA WITH 5 CHANNELS COMPETITION/Striatum D1 /Striatum D1 /StrSat ==
  In1 : Inport
  Fcn : Fcn  Expr=u^(1/nu_str)
  "Leaky-Integrator Striatum D1 " : ZeroPole  Zeros=[]  Poles=[-1/teta]  Gain=[1.5/teta]
  Sigmoidal MF : fuzblock/Membership  Functions/Sigmoidal MF  a=alpha_str  c=beta_str
      settings: SourceProductName=Fuzzy Logic Toolbox  SourceProductBaseCode=FL
  Out1 : Outport
  wires:
  Fcn/1 -> Out1/1
  Sigmoidal MF/1 -> Fcn/1
  "Leaky-Integrator Striatum D1 "/1 -> Sigmoidal MF/1
  In1/1 -> "Leaky-Integrator Striatum D1 "/1

== system ExtensionSimulation1var_5/BASAL GANGLIA WITH 5 CHANNELS COMPETITION/Striatum D1 /Striatum D1 /StrSat1 ==
  In1 : Inport
  Fcn : Fcn  Expr=u^(1/nu_str)
  "Leaky-Integrator Striatum D1 " : ZeroPole  Zeros=[]  Poles=[-1/teta]  Gain=[1.5/teta]
  Sigmoidal MF : fuzblock/Membership  Functions/Sigmoidal MF  a=alpha_str  c=beta_str
      settings: SourceProductName=Fuzzy Logic Toolbox  SourceProductBaseCode=FL
  Out1 : Outport
  wires:
  Fcn/1 -> Out1/1
  Sigmoidal MF/1 -> Fcn/1
  "Leaky-Integrator Striatum D1 "/1 -> Sigmoidal MF/1
  In1/1 -> "Leaky-Integrator Striatum D1 "/1

== system ExtensionSimulation1var_5/BASAL GANGLIA WITH 5 CHANNELS COMPETITION/Striatum D1 /Striatum D1 /StrSat2 ==
  In1 : Inport
  Fcn : Fcn  Expr=u^(1/nu_str)
  "Leaky-Integrator Striatum D1 " : ZeroPole  Zeros=[]  Poles=[-1/teta]  Gain=[1.5/teta]
  Sigmoidal MF : fuzblock/Membership  Functions/Sigmoidal MF  a=alpha_str  c=beta_str
      settings: SourceProductName=Fuzzy Logic Toolbox  SourceProductBaseCode=FL
  Out1 : Outport
  wires:
  Fcn/1 -> Out1/1
  Sigmoidal MF/1 -> Fcn/1
  "Leaky-Integrator Striatum D1 "/1 -> Sigmoidal MF/1
  In1/1 -> "Leaky-Integrator Striatum D1 "/1

== system ExtensionSimulation1var_5/BASAL GANGLIA WITH 5 CHANNELS COMPETITION/Striatum D1 /Striatum D1 /StrSat3 ==
  In1 : Inport
  Fcn : Fcn  Expr=u^(1/nu_str)
  "Leaky-Integrator Striatum D1 " : ZeroPole  Zeros=[]  Poles=[-1/teta]  Gain=[1.5/teta]
  Sigmoidal MF : fuzblock/Membership  Functions/Sigmoidal MF  a=alpha_str  c=beta_str
      settings: SourceProductName=Fuzzy Logic Toolbox  SourceProductBaseCode=FL
  Out1 : Outport
  wires:
  Fcn/1 -> Out1/1
  Sigmoidal MF/1 -> Fcn/1
  "Leaky-Integrator Striatum D1 "/1 -> Sigmoidal MF/1
  In1/1 -> "Leaky-Integrator Striatum D1 "/1

== system ExtensionSimulation1var_5/BASAL GANGLIA WITH 5 CHANNELS COMPETITION/Striatum D1 /Striatum D1 /StrSat4 ==
  In1 : Inport
  Fcn : Fcn  Expr=u^(1/nu_str)
  "Leaky-Integrator Striatum D1 " : ZeroPole  Zeros=[]  Poles=[-1/teta]  Gain=[1.5/teta]
  Sigmoidal MF : fuzblock/Membership  Functions/Sigmoidal MF  a=alpha_str  c=beta_str
      settings: SourceProductName=Fuzzy Logic Toolbox  SourceProductBaseCode=FL
  Out1 : Outport
  wires:
  Fcn/1 -> Out1/1
  Sigmoidal MF/1 -> Fcn/1
  "Leaky-Integrator Striatum D1 "/1 -> Sigmoidal MF/1
  In1/1 -> "Leaky-Integrator Striatum D1 "/1

== system ExtensionSimulation1var_5/BASAL GANGLIA WITH 5 CHANNELS COMPETITION/Striatum D2/Striatum D2 /StrSat ==
  In1 : Inport
  Fcn : Fcn  Expr=u^(1/nu_str)
  "Leaky-Integrator Striatum D1 " : ZeroPole  Zeros=[]  Poles=[-1/teta]  Gain=[1.5/teta]
  Sigmoidal MF : fuzblock/Membership  Functions/Sigmoidal MF  a=alpha_str  c=beta_str
      settings: SourceProductName=Fuzzy Logic Toolbox  SourceProductBaseCode=FL
  Out1 : Outport
  wires:
  Fcn/1 -> Out1/1
  Sigmoidal MF/1 -> Fcn/1
  "Leaky-Integrator Striatum D1 "/1 -> Sigmoidal MF/1
  In1/1 -> "Leaky-Integrator Striatum D1 "/1

== system ExtensionSimulation1var_5/BASAL GANGLIA WITH 5 CHANNELS COMPETITION/Striatum D2/Striatum D2 /StrSat1 ==
  In1 : Inport
  Fcn : Fcn  Expr=u^(1/nu_str)
  "Leaky-Integrator Striatum D1 " : ZeroPole  Zeros=[]  Poles=[-1/teta]  Gain=[1.5/teta]
  Sigmoidal MF : fuzblock/Membership  Functions/Sigmoidal MF  a=alpha_str  c=beta_str
      settings: SourceProductName=Fuzzy Logic Toolbox  SourceProductBaseCode=FL
  Out1 : Outport
  wires:
  Fcn/1 -> Out1/1
  Sigmoidal MF/1 -> Fcn/1
  "Leaky-Integrator Striatum D1 "/1 -> Sigmoidal MF/1
  In1/1 -> "Leaky-Integrator Striatum D1 "/1

== system ExtensionSimulation1var_5/BASAL GANGLIA WITH 5 CHANNELS COMPETITION/Striatum D2/Striatum D2 /StrSat2 ==
  In1 : Inport
  Fcn : Fcn  Expr=u^(1/nu_str)
  "Leaky-Integrator Striatum D1 " : ZeroPole  Zeros=[]  Poles=[-1/teta]  Gain=[1.5/teta]
  Sigmoidal MF : fuzblock/Membership  Functions/Sigmoidal MF  a=alpha_str  c=beta_str
      settings: SourceProductName=Fuzzy Logic Toolbox  SourceProductBaseCode=FL
  Out1 : Outport
  wires:
  Fcn/1 -> Out1/1
  Sigmoidal MF/1 -> Fcn/1
  "Leaky-Integrator Striatum D1 "/1 -> Sigmoidal MF/1
  In1/1 -> "Leaky-Integrator Striatum D1 "/1

== system ExtensionSimulation1var_5/BASAL GANGLIA WITH 5 CHANNELS COMPETITION/Striatum D2/Striatum D2 /StrSat3 ==
  In1 : Inport
  Fcn : Fcn  Expr=u^(1/nu_str)
  "Leaky-Integrator Striatum D1 " : ZeroPole  Zeros=[]  Poles=[-1/teta]  Gain=[1.5/teta]
  Sigmoidal MF : fuzblock/Membership  Functions/Sigmoidal MF  a=alpha_str  c=beta_str
      settings: SourceProductName=Fuzzy Logic Toolbox  SourceProductBaseCode=FL
  Out1 : Outport
  wires:
  Fcn/1 -> Out1/1
  Sigmoidal MF/1 -> Fcn/1
  "Leaky-Integrator Striatum D1 "/1 -> Sigmoidal MF/1
  In1/1 -> "Leaky-Integrator Striatum D1 "/1

== system ExtensionSimulation1var_5/BASAL GANGLIA WITH 5 CHANNELS COMPETITION/Striatum D2/Striatum D2 /StrSat4 ==
  In1 : Inport
  Fcn : Fcn  Expr=u^(1/nu_str)
  "Leaky-Integrator Striatum D1 " : ZeroPole  Zeros=[]  Poles=[-1/teta]  Gain=[1.5/teta]
  Sigmoidal MF : fuzblock/Membership  Functions/Sigmoidal MF  a=alpha_str  c=beta_str
      settings: SourceProductName=Fuzzy Logic Toolbox  SourceProductBaseCode=FL
  Out1 : Outport
  wires:
  Fcn/1 -> Out1/1
  Sigmoidal MF/1 -> Fcn/1
  "Leaky-Integrator Striatum D1 "/1 -> Sigmoidal MF/1
  In1/1 -> "Leaky-Integrator Striatum D1 "/1

== system ExtensionSimulation1var_5/BASAL GANGLIA WITH 5 CHANNELS COMPETITION/SubThalamic Nuclei/SubThalamic Nucleus (STN) /StnSat ==
  In1 : Inport
  Fcn : Fcn  Expr=u^(1/nu_stn)
  "Leaky-Integrator Striatum D1 " : ZeroPole  Zeros=[]  Poles=[-1/teta]  Gain=[1.5/teta]
  Sigmoidal MF : fuzblock/Membership  Functions/Sigmoidal MF  a=alpha_stn  c=beta_stn
      settings: SourceProductName=Fuzzy Logic Toolbox  SourceProductBaseCode=FL
  Out1 : Outport
  wires:
  Fcn/1 -> Out1/1
  Sigmoidal MF/1 -> Fcn/1
  "Leaky-Integrator Striatum D1 "/1 -> Sigmoidal MF/1
  In1/1 -> "Leaky-Integrator Striatum D1 "/1

== system ExtensionSimulation1var_5/BASAL GANGLIA WITH 5 CHANNELS COMPETITION/SubThalamic Nuclei/SubThalamic Nucleus (STN) /StnSat1 ==
  In1 : Inport
  Fcn : Fcn  Expr=u^(1/nu_stn)
  "Leaky-Integrator Striatum D1 " : ZeroPole  Zeros=[]  Poles=[-1/teta]  Gain=[1.5/teta]
  Sigmoidal MF : fuzblock/Membership  Functions/Sigmoidal MF  a=alpha_stn  c=beta_stn
      settings: SourceProductName=Fuzzy Logic Toolbox  SourceProductBaseCode=FL
  Out1 : Outport
  wires:
  Fcn/1 -> Out1/1
  Sigmoidal MF/1 -> Fcn/1
  "Leaky-Integrator Striatum D1 "/1 -> Sigmoidal MF/1
  In1/1 -> "Leaky-Integrator Striatum D1 "/1

== system ExtensionSimulation1var_5/BASAL GANGLIA WITH 5 CHANNELS COMPETITION/SubThalamic Nuclei/SubThalamic Nucleus (STN) /StnSat2 ==
  In1 : Inport
  Fcn : Fcn  Expr=u^(1/nu_stn)
  "Leaky-Integrator Striatum D1 " : ZeroPole  Zeros=[]  Poles=[-1/teta]  Gain=[1.5/teta]
  Sigmoidal MF : fuzblock/Membership  Functions/Sigmoidal MF  a=alpha_stn  c=beta_stn
      settings: SourceProductName=Fuzzy Logic Toolbox  SourceProductBaseCode=FL
  Out1 : Outport
  wires:
  Fcn/1 -> Out1/1
  Sigmoidal MF/1 -> Fcn/1
  "Leaky-Integrator Striatum D1 "/1 -> Sigmoidal MF/1
  In1/1 -> "Leaky-Integrator Striatum D1 "/1

== system ExtensionSimulation1var_5/BASAL GANGLIA WITH 5 CHANNELS COMPETITION/SubThalamic Nuclei/SubThalamic Nucleus (STN) /StnSat3 ==
  In1 : Inport
  Fcn : Fcn  Expr=u^(1/nu_stn)
  "Leaky-Integrator Striatum D1 " : ZeroPole  Zeros=[]  Poles=[-1/teta]  Gain=[1.5/teta]
  Sigmoidal MF : fuzblock/Membership  Functions/Sigmoidal MF  a=alpha_stn  c=beta_stn
      settings: SourceProductName=Fuzzy Logic Toolbox  SourceProductBaseCode=FL
  Out1 : Outport
  wires:
  Fcn/1 -> Out1/1
  Sigmoidal MF/1 -> Fcn/1
  "Leaky-Integrator Striatum D1 "/1 -> Sigmoidal MF/1
  In1/1 -> "Leaky-Integrator Striatum D1 "/1

== system ExtensionSimulation1var_5/BASAL GANGLIA WITH 5 CHANNELS COMPETITION/SubThalamic Nuclei/SubThalamic Nucleus (STN) /StnSat4 ==
  In1 : Inport
  Fcn : Fcn  Expr=u^(1/nu_stn)
  "Leaky-Integrator Striatum D1 " : ZeroPole  Zeros=[]  Poles=[-1/teta]  Gain=[1.5/teta]
  Sigmoidal MF : fuzblock/Membership  Functions/Sigmoidal MF  a=alpha_stn  c=beta_stn
      settings: SourceProductName=Fuzzy Logic Toolbox  SourceProductBaseCode=FL
  Out1 : Outport
  wires:
  Fcn/1 -> Out1/1
  Sigmoidal MF/1 -> Fcn/1
  "Leaky-Integrator Striatum D1 "/1 -> Sigmoidal MF/1
  In1/1 -> "Leaky-Integrator Striatum D1 "/1

== matlab function ExtensionSimulation1var_5/BASAL GANGLIA WITH 5 CHANNELS COMPETITION/Striatum D2/MATLAB Function ==
  data: ch_in input; ch_out output; w_inhib input
function ch_out = recurrent_inh(ch_in, w_inhib)
    
   ch_out = zeros(1,5);
   for ii = 1:5
        
        kronD = ones(1,5);
        kronD(ii) = 0;
        ch_out(ii) = ch_in(ii) - w_inhib*(sum(ch_in.*kronD'));

   end
end

== matlab function ExtensionSimulation1var_5/BASAL GANGLIA WITH 5 CHANNELS COMPETITION/Striatum D1 /MATLAB Function ==
  data: ch_in input; ch_out output; w_inhib input
function ch_out = recurrent_inh(ch_in, w_inhib)
    
   ch_out = zeros(1,5);
   for ii = 1:5
        
        kronD = ones(1,5);
        kronD(ii) = 0;
        ch_out(ii) = ch_in(ii) - w_inhib*(sum(ch_in.*kronD'));

   end
end
